simulink model "dynamiczny_dyskretny"  (R2017b)
settings: Solver=VariableStepAuto  StartTime=0.0  StopTime=time  RelTol=1e-3
values from neighbouring files (symbols this model uses):
  alfa1 = -0.9    [params.m]
  alfa2 = 1.37    [params.m]
  alfa3 = -1.95    [params.m]
  alfa4 = 0.05    [params.m]
  DelayValue = 1    [params.m]
  K = 5    [params.m]
  StartDelay = 5    [params.m]
  StartValue = 0    [params.m]
  T = 1    [params.m]
  T1 = 10    [params.m]
  T2 = 6    [params.m]
settings Model: Creator=Tomek  LastModifiedBy=Tomek

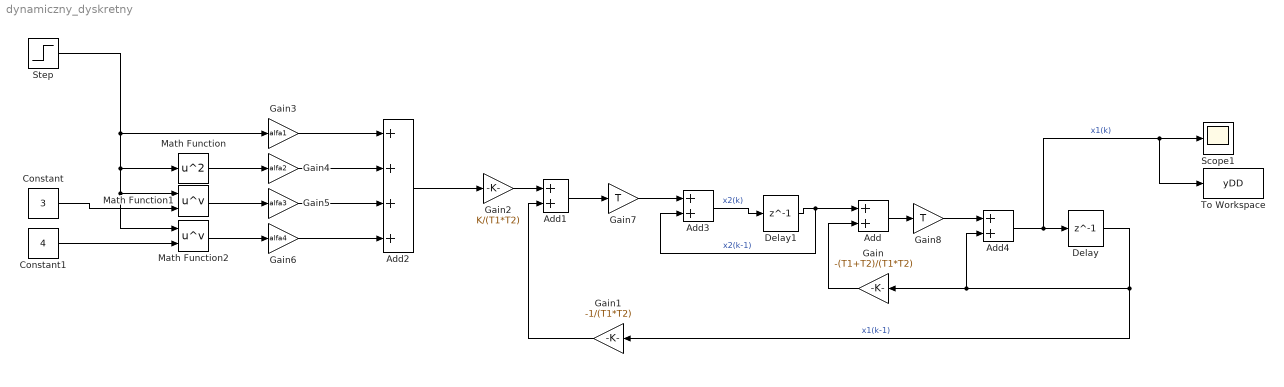
== system dynamiczny_dyskretny ==
  Add{,1,3..4} (4 alike) : Sum
  Add2 : Sum  Inputs=++++
  Constant : Constant  Value=3
  Constant1 : Constant  Value=4
  Delay : Delay  DelayLength=1  SampleTime=T
  Delay1 : Delay  DelayLength=1  SampleTime=T
  Gain : Gain  Gain=-(T1+T2)/(T1*T2)
  Gain1 : Gain  Gain=-1/(T1*T2)
  Gain2 : Gain  Gain=K/(T1*T2)
  Gain3 : Gain  Gain=alfa1
  Gain4 : Gain  Gain=alfa2
  Gain5 : Gain  Gain=alfa3
  Gain6 : Gain  Gain=alfa4
  Gain7 : Gain  Gain=T
  Gain8 : Gain  Gain=T
  Math Function : Math  Operator=square  SaturateOnIntegerOverflow=on
  Math Function1 : Math  Operator=pow  SaturateOnIntegerOverflow=on
  Math Function2 : Math  Operator=pow  SaturateOnIntegerOverflow=on
  Scope1 : Scope
  Step : Step  Time=StartDelay  Before=StartValue  After=DelayValue  SampleTime=0
  To Workspace : ToWorkspace  VariableName=yDD  SaveFormat=Timeseries  SampleTime=-1
  wires:
  Constant/1 -> Math Function1/2
  Gain4/1 -> Add2/2
  Constant1/1 -> Math Function2/2
  Step/1 -> Math Function2/1, Math Function1/1, Math Function/1, Gain3/1
  Add2/1 -> Gain2/1
  Math Function2/1 -> Gain6/1
  Math Function1/1 -> Gain5/1
  Gain1/1 -> Add1/2
  Gain/1 -> Add/2
  Math Function/1 -> Gain4/1
  Gain3/1 -> Add2/1
  Gain2/1 -> Add1/1
  Add3/1 -> Delay1/1  "x2(k)"
  Delay1/1 -> Add3/2, Add/1  "x2(k-1)"
  Delay/1 -> Gain1/1, Add4/2, Gain/1  "x1(k-1)"
  Gain5/1 -> Add2/3
  Gain6/1 -> Add2/4
  Add4/1 -> To Workspace/1, Scope1/1, Delay/1  "x1(k)"
  Add1/1 -> Gain7/1
  Gain7/1 -> Add3/1
  Add/1 -> Gain8/1
  Gain8/1 -> Add4/1
